simulink model "FINAL_BOARD_6437_EVM"  (Simulink 7.4)
settings: Solver=FixedStepDiscrete  StartTime=0.0  StopTime=inf  FixedStep=1/8000  RelTol=1e-3
undefined symbols (not defined in the file): M, N, SW4, sz
libraries: vipmisc x9, davincilib x6, viptransforms x3, vipconversions x3, vipgeotforms x3, dm6437evmlib x1, idelinklib_tgtpref x1, vipsrcs x1
settings Model: Creator=dsp0105  LastModifiedBy=mattwharper
settings SolverCC: PositivePriorityOrder=on
settings DataIOCC: SaveOutput=off  SaveTime=off
settings HardwareCC: ProdBitPerLong=40  ProdIntDivRoundTo=Zero  ProdEndianess=LittleEndian  ProdHWDeviceType=Texas Instruments->C6000
settings RTWCC: SystemTargetFile=ccslink_grt.tlc  GenCodeOnly=on  GenerateMakefile=off  TemplateMakefile=none  Description=Embedded IDE Link (for use with Texas Instruments(TM) Code Composer Studio(TM)) GRT code generation  ProcessScript=ccslink_grt_make_rtw_hook
settings GRTTgtLinkCCS: TargetFcnLib=ansi_tfl_table_tmw.mat  TargetFunctionLibrary=ANSI_C  UtilityFuncGeneration=Auto  ERTMultiwordTypeDef=System defined  ERTMultiwordLength=256  MultiwordLength=2048  GenerateFullHeader=on  GenerateSampleERTMain=off  GenerateTestInterfaces=off  IsPILTarget=off  ModelReferenceCompliant=on  ParMdlRefBuildCompliant=off  CompOptLevelCompliant=off  IncludeMdlTerminateFcn=on  GeneratePreprocessorConditionals=Disable all  CombineOutputUpdateFcns=off  SuppressErrorStatus=off  ERTFirstTimeCompliant=off  IncludeFileDelimiter=Auto  ERTCustomFileBanners=off  SupportAbsoluteTime=on  LogVarNameModifier=rt_  MatFileLogging=off  MultiInstanceERTCode=off  SupportNonFinite=on  SupportComplex=on  PurelyIntegerCode=off  SupportContinuousTime=on  SupportNonInlinedSFcns=on  SupportVariableSizeSignals=off  EnableShiftOperators=on  ParenthesesLevel=Nominal  PortableWordSizes=off  ModelStepFunctionPrototypeControlCompliant=off  CPPClassGenCompliant=off  AutosarCompliant=off  GenerateASAP2=off  ExtMode=off  ExtModeTransport=0  ExtModeStaticAlloc=off  ExtModeStaticAllocSize=1000000  ExtModeTesting=off  ExtModeMexFile=ext_comm  ExtModeIntrfLevel=Level1  RTWCAPISignals=off  RTWCAPIParams=off  RTWCAPIStates=off  exportCCSObj=on  ccsObjName=CCS_Obj  exportIDEObj=on  ideObjName=CCS_Obj  oldideObjName=CCS_Obj  ideObjTimeout=10  oldideObjTimeout=10  ideObjBuildTimeout=1000  oldideObjBuildTimeout=1000  ProfileGenCode=off  profileBy=Tasks  ProfileNumSamples=100  InlineDSPBlks=off  projectOptions=Custom  debugCompilerOptions="-g -d\"_DEBUG\""  releaseCompilerOptions=-o2  customCompilerOptions=-o2-q  compilerOptionsStr=-o2-q  getCompilerOptions=off  getLinkerOptions=off  systemStackSize=8192  buildAction=Build_and_execute  overrunNotificationMethod=None  overrunNotificationFcn=myfunction  oldoverrunNotificationFcn=myfunction  DiagnosticActions=warning

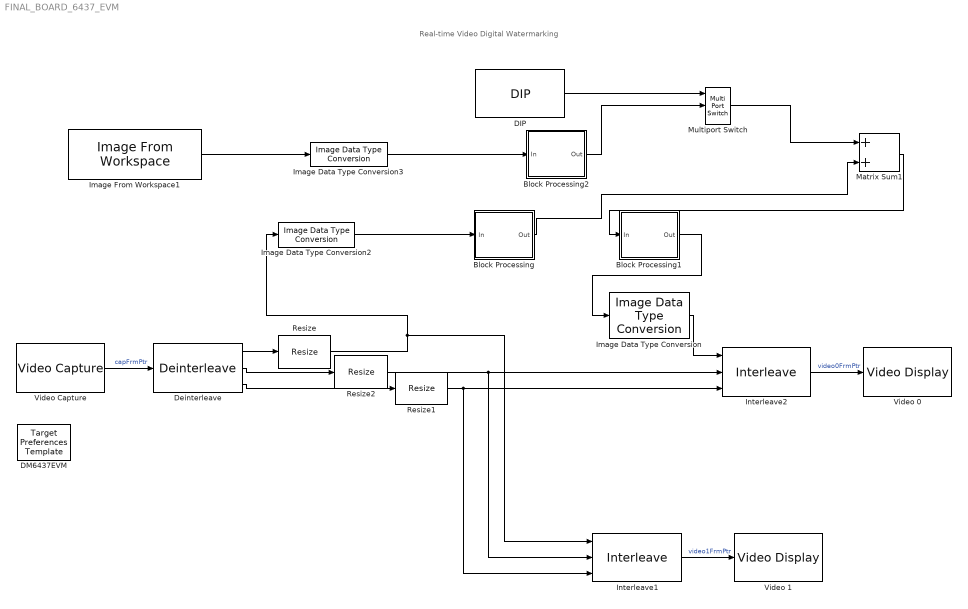
== system FINAL_BOARD_6437_EVM ==
  note: Real-time Video Digital Watermarking
  Block Processing : Subsystem  DialogController=vipDDGCreate  DialogControllerArgs=DataTag0  TreatAsAtomicUnit=on  mask(Block Processing){NumI=1, NumO=1, Blocksize={[8 8]}, Overlapsize={[0 0]}, Traverse=Row-wise}
      mask prompts: NumI "Number of inputs:"; NumO "Number of outputs:"; Blocksize "Block size:"; Overlapsize "Overlap size:"; Traverse "Order of traversing:"
      mask help:
      | Repeats a user-specified operation on submatrices of the input matrix.
      |
      | This block extracts submatrices of a user-specified size from the input matrix. It sends each submatrix to a subsystem for processing, and then reassembles each subsystem output into the output matrix.
      |
      | Use the Block size and Overlap parameters to specify the size and overlap of each submatrix in cell array format.
      mask init:
      | errmsg = vipblkblockproc(gcbh, NumI, NumO, Blocksize, Overlapsize, Traverse);
      | error(errmsg);
      settings: CopyFcn=set_param(gcb,'LinkStatus','none');
      mask Help: eval('helpview(fullfile(docroot,''toolbox'',''vipblks'',''vipblks.map''),''vipblockprocessing'')');
      mask StyleString: edit,edit,edit,edit,popup(Row-wise|Column-wise)
      mask Display: disp('Block\n Processing');
  Block Processing1 : Subsystem  DialogController=vipDDGCreate  DialogControllerArgs=DataTag2  TreatAsAtomicUnit=on  mask(Block Processing){NumI=1, NumO=1, Blocksize={[8 8]}, Overlapsize={[0 0]}, Traverse=Row-wise}
      mask prompts: NumI "Number of inputs:"; NumO "Number of outputs:"; Blocksize "Block size:"; Overlapsize "Overlap size:"; Traverse "Order of traversing:"
      mask help:
      | Repeats a user-specified operation on submatrices of the input matrix.
      |
      | This block extracts submatrices of a user-specified size from the input matrix. It sends each submatrix to a subsystem for processing, and then reassembles each subsystem output into the output matrix.
      |
      | Use the Block size and Overlap parameters to specify the size and overlap of each submatrix in cell array format.
      mask init:
      | errmsg = vipblkblockproc(gcbh, NumI, NumO, Blocksize, Overlapsize, Traverse);
      | error(errmsg);
      settings: CopyFcn=set_param(gcb,'LinkStatus','none');
      mask Help: eval('helpview(fullfile(docroot,''toolbox'',''vipblks'',''vipblks.map''),''vipblockprocessing'')');
      mask StyleString: edit,edit,edit,edit,popup(Row-wise|Column-wise)
      mask Display: disp('Block\n Processing');
  Block Processing2 : Subsystem  DialogController=vipDDGCreate  DialogControllerArgs=DataTag4  TreatAsAtomicUnit=on  mask(Block Processing){NumI=1, NumO=1, Blocksize={[8 8]}, Overlapsize={[0 0]}, Traverse=Row-wise}
      mask prompts: NumI "Number of inputs:"; NumO "Number of outputs:"; Blocksize "Block size:"; Overlapsize "Overlap size:"; Traverse "Order of traversing:"
      mask help:
      | Repeats a user-specified operation on submatrices of the input matrix.
      |
      | This block extracts submatrices of a user-specified size from the input matrix. It sends each submatrix to a subsystem for processing, and then reassembles each subsystem output into the output matrix.
      |
      | Use the Block size and Overlap parameters to specify the size and overlap of each submatrix in cell array format.
      mask init:
      | errmsg = vipblkblockproc(gcbh, NumI, NumO, Blocksize, Overlapsize, Traverse);
      | error(errmsg);
      settings: CopyFcn=set_param(gcb,'LinkStatus','none');
      mask Help: eval('helpview(fullfile(docroot,''toolbox'',''vipblks'',''vipblks.map''),''vipblockprocessing'')');
      mask StyleString: edit,edit,edit,edit,popup(Row-wise|Column-wise)
      mask Display: disp('Block\n Processing');
  DIP : dm6437evmlib/DIP  SystemSampleTime=-1  dipSwitch=SW4(0)  sampleTime=1
  DM6437EVM : idelinklib_tgtpref/Target Preferences Template  Tag=ccslinktgtpref  SystemSampleTime=-1
  Deinterleave : davincilib/Deinterleave  SystemSampleTime=-1
  Image Data Type Conversion : vipconversions/Image Data Type Conversion  outDT=uint8  isSigned=on  wordLen=16  numFracBits=0
  Image Data Type Conversion2 : vipconversions/Image Data Type Conversion  outDT=single  isSigned=on  wordLen=16  numFracBits=0
  Image Data Type Conversion3 : vipconversions/Image Data Type Conversion  outDT=single  isSigned=on  wordLen=16  numFracBits=0
  Image From Workspace1 : vipsrcs/Image From Workspace  Tag=vipblks_nd  SystemSampleTime=-1  ImageValue=h  Ts=inf  imagePorts=One multidimensional signal  ImageDataType=Inherit from 'Value'  Signed=on  WordLength=16  sdImageDataType=sfix(16)  FractionLengthMode=User-defined  FractionLength=15  OutPortLabels=R|G|B
  Interleave1 : davincilib/Interleave  SystemSampleTime=-1  outPitch=32
  Interleave2 : davincilib/Interleave  SystemSampleTime=-1  outPitch=32
  Matrix Sum1 : Sum  OutDataType=sfix(16)  OutScaling=2^-10
  Multiport Switch : MultiPortSwitch  Inputs=2  OutDataType=fixdt(1, 16)  OutScaling=2^0
  Resize : vipgeotforms/Resize  DialogController=vipDDGCreate  DialogControllerArgs=DataTag7  specify=Number of output rows and columns  rfactor=[176 128]  outCols=25  outRows=25  outRowsCols=[176 128]  interp_method=Bilinear  antialias=off  useROI=off  roiFlag=off  prodOutputMode=Binary point scaling  prodOutputWordLength=32  prodOutputFracLength=10  roundingMode=Nearest  overflowMode=on
  Resize1 : vipgeotforms/Resize  DialogController=vipDDGCreate  DialogControllerArgs=DataTag8  specify=Number of output rows and columns  rfactor=[88 128]  outCols=25  outRows=25  outRowsCols=[88 128]  interp_method=Nearest neighbor  antialias=off  useROI=off  roiFlag=off  prodOutputMode=Binary point scaling  prodOutputWordLength=32  prodOutputFracLength=10  roundingMode=Nearest  overflowMode=on
  Resize2 : vipgeotforms/Resize  DialogController=vipDDGCreate  DialogControllerArgs=DataTag9  specify=Number of output rows and columns  rfactor=[88 128]  outCols=25  outRows=25  outRowsCols=[88 128]  interp_method=Nearest neighbor  antialias=off  useROI=off  roiFlag=off  prodOutputMode=Binary point scaling  prodOutputWordLength=32  prodOutputFracLength=10  roundingMode=Nearest  overflowMode=on
  Video 0 : davincilib/Video Display  videoWindow=Video0  video0Position=[180, 0,360, 480]  video1LocSrc=Specify via dialog  video1Location=[320, 200, 152, 100]  hZoom=2x  vZoom=2x  videoEnablePort=off  videoDisplayMode=NTSC  avOutput=Composite  hExpansion=off  vExpansion=off
  Video 1 : davincilib/Video Display  videoWindow=Video1  video0Position=180, 0,360, 480]  video1LocSrc=Specify via dialog  video1Location=[0, 240, 360, 240]  hZoom=2x  vZoom=2x  videoEnablePort=off  videoDisplayMode=NTSC  avOutput=Composite  hExpansion=off  vExpansion=off
  Video Capture : davincilib/Video Capture  videoCaptureMode=NTSC  avInput=Composite  sampleTime=-1
  wires:
  Video Capture/1 -> Deinterleave/1  "capFrmPtr"
  Interleave2/1 -> Video 0/1  "video0FrmPtr"
  Image Data Type Conversion/1 -> Interleave2/1
  Deinterleave/3 -> Resize1/1
  Deinterleave/2 -> Resize2/1
  Deinterleave/1 -> Resize/1
  Block Processing1/1(Out) -> Image Data Type Conversion/1
  Interleave1/1 -> Video 1/1  "video1FrmPtr"
  Multiport Switch/1 -> Matrix Sum1/1
  Block Processing2/1(Out) -> Multiport Switch/2
  DIP/1 -> Multiport Switch/1
  Matrix Sum1/1 -> Block Processing1/1(In)
  Block Processing/1(Out) -> Matrix Sum1/2
  Image From Workspace1/1 -> Image Data Type Conversion3/1
  Image Data Type Conversion3/1 -> Block Processing2/1(In)
  Image Data Type Conversion2/1 -> Block Processing/1(In)
  Resize/1 -> Interleave1/1, Image Data Type Conversion2/1
  Resize2/1 -> Interleave2/2, Interleave1/2
  Resize1/1 -> Interleave2/3, Interleave1/3

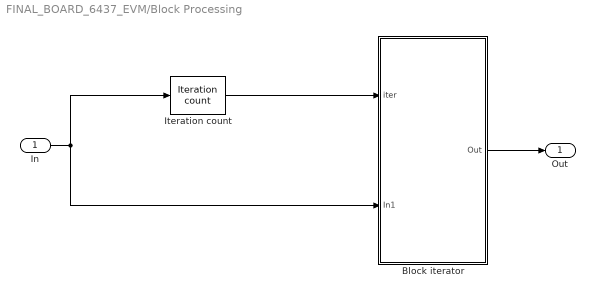
== system FINAL_BOARD_6437_EVM/Block Processing ==
  In : Inport  OutDataType=sfix(16)  OutScaling=2^0
  Block iterator : Subsystem
      settings: CopyFcn=set_param(gcb,'ReferenceBlock','');
  Iteration count : vipmisc/Iteration count  blksize=Blocksize{1}  ovlpsize=Overlapsize{1}
  Out : Outport  OutDataType=sfix(16)  OutScaling=2^0
  wires:
  Iteration count/1 -> Block iterator/1(iter)
  In/1 -> Iteration count/1, Block iterator/2(In1)
  Block iterator/1(Out) -> Out/1

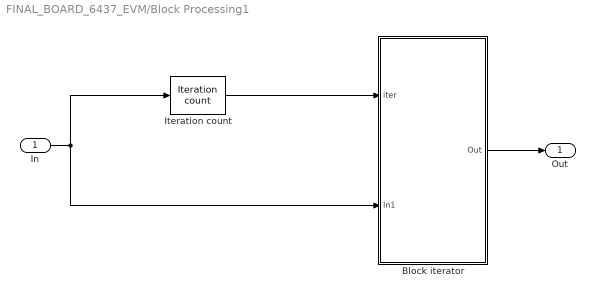
== system FINAL_BOARD_6437_EVM/Block Processing1 ==
  In : Inport  OutDataType=sfix(16)  OutScaling=2^0
  Block iterator : Subsystem
      settings: CopyFcn=set_param(gcb,'ReferenceBlock','');
  Iteration count : vipmisc/Iteration count  blksize=Blocksize{1}  ovlpsize=Overlapsize{1}
  Out : Outport  OutDataType=sfix(16)  OutScaling=2^0
  wires:
  Iteration count/1 -> Block iterator/1(iter)
  In/1 -> Iteration count/1, Block iterator/2(In1)
  Block iterator/1(Out) -> Out/1

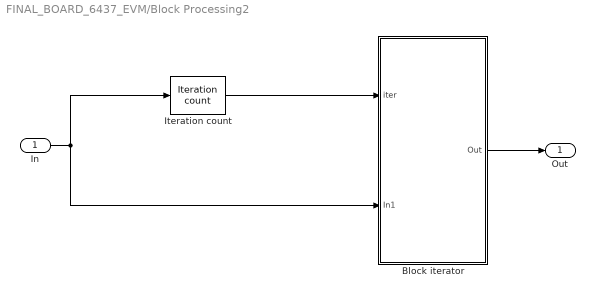
== system FINAL_BOARD_6437_EVM/Block Processing2 ==
  In : Inport  OutDataType=sfix(16)  OutScaling=2^0
  Block iterator : Subsystem
      settings: CopyFcn=set_param(gcb,'ReferenceBlock','');
  Iteration count : vipmisc/Iteration count  blksize=Blocksize{1}  ovlpsize=Overlapsize{1}
  Out : Outport  OutDataType=sfix(16)  OutScaling=2^0
  wires:
  Iteration count/1 -> Block iterator/1(iter)
  In/1 -> Iteration count/1, Block iterator/2(In1)
  Block iterator/1(Out) -> Out/1

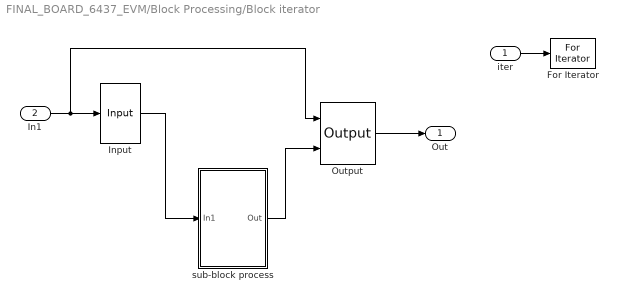
== system FINAL_BOARD_6437_EVM/Block Processing/Block iterator ==
  iter : Inport  OutDataType=sfix(16)  OutScaling=2^0
  In1 : Inport  Port=2  OutDataType=sfix(16)  OutScaling=2^0
  For Iterator : ForIterator  IterationSource=external  IterationLimit=(sz(1)/M)*(sz(2)/N)  ShowIterationPort=off  IndexMode=Zero-based  IterationVariableDataType=double
  Input : vipmisc/Input  SystemSampleTime=-1  Blocksize=Blocksize{1}  Overlapsize=Overlapsize{1}  tverse=Row-wise
  Output : vipmisc/Output  SystemSampleTime=-1  Blocksize=Blocksize{1}  Overlapsize=Overlapsize{1}  tverse=Row-wise
  sub-block process : Subsystem
  Out : Outport  OutDataType=sfix(16)  OutScaling=2^0
  wires:
  iter/1 -> For Iterator/1
  In1/1 -> Output/1, Input/1
  Output/1 -> Out/1
  sub-block process/1(Out) -> Output/2
  Input/1 -> sub-block process/1(In1)

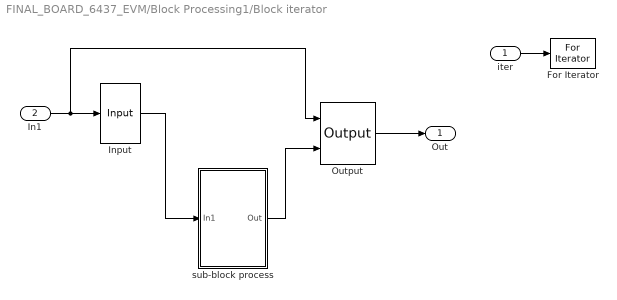
== system FINAL_BOARD_6437_EVM/Block Processing1/Block iterator ==
  iter : Inport  OutDataType=sfix(16)  OutScaling=2^0
  In1 : Inport  Port=2  OutDataType=sfix(16)  OutScaling=2^0
  For Iterator : ForIterator  IterationSource=external  IterationLimit=(sz(1)/M)*(sz(2)/N)  ShowIterationPort=off  IndexMode=Zero-based  IterationVariableDataType=double
  Input : vipmisc/Input  SystemSampleTime=-1  Blocksize=Blocksize{1}  Overlapsize=Overlapsize{1}  tverse=Row-wise
  Output : vipmisc/Output  SystemSampleTime=-1  Blocksize=Blocksize{1}  Overlapsize=Overlapsize{1}  tverse=Row-wise
  sub-block process : Subsystem
  Out : Outport  OutDataType=sfix(16)  OutScaling=2^0
  wires:
  iter/1 -> For Iterator/1
  In1/1 -> Output/1, Input/1
  Output/1 -> Out/1
  sub-block process/1(Out) -> Output/2
  Input/1 -> sub-block process/1(In1)

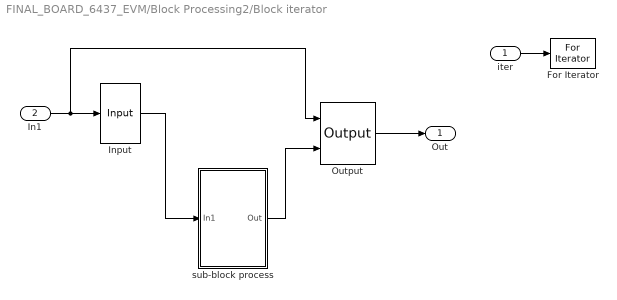
== system FINAL_BOARD_6437_EVM/Block Processing2/Block iterator ==
  iter : Inport  OutDataType=sfix(16)  OutScaling=2^0
  In1 : Inport  Port=2  OutDataType=sfix(16)  OutScaling=2^0
  For Iterator : ForIterator  IterationSource=external  IterationLimit=(sz(1)/M)*(sz(2)/N)  ShowIterationPort=off  IndexMode=Zero-based  IterationVariableDataType=double
  Input : vipmisc/Input  SystemSampleTime=-1  Blocksize=Blocksize{1}  Overlapsize=Overlapsize{1}  tverse=Row-wise
  Output : vipmisc/Output  SystemSampleTime=-1  Blocksize=Blocksize{1}  Overlapsize=Overlapsize{1}  tverse=Row-wise
  sub-block process : Subsystem
  Out : Outport  OutDataType=sfix(16)  OutScaling=2^0
  wires:
  iter/1 -> For Iterator/1
  In1/1 -> Output/1, Input/1
  Output/1 -> Out/1
  sub-block process/1(Out) -> Output/2
  Input/1 -> sub-block process/1(In1)

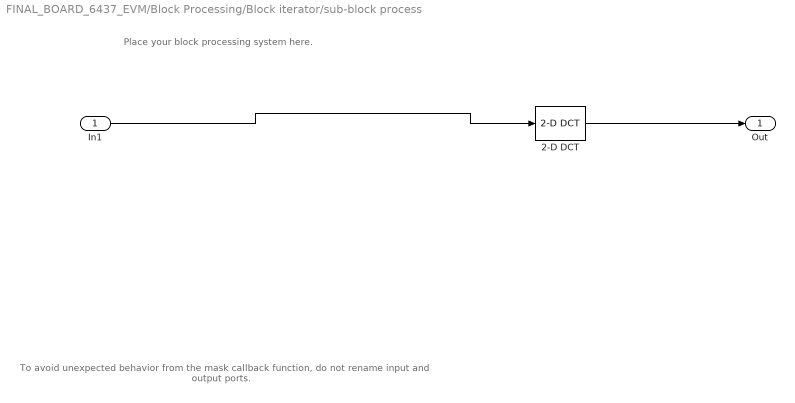
== system FINAL_BOARD_6437_EVM/Block Processing/Block iterator/sub-block process ==
  note: To avoid unexpected behavior from the mask
      | callback function, do not rename input and output ports.
  note: Place your block
      | processing system here.
  In1 : Inport  OutDataType=sfix(16)  OutScaling=2^0
  2-D DCT : viptransforms/2-D DCT  DialogController=dspDDGCreate  DialogControllerArgs=DataTag1  CompMethod=Table lookup  Dimension=0  TableOpt=Speed  BitRevOrder=off  SkipNorm=off  roundingMode=Floor  overflowMode=off
  Out : Outport  OutDataType=sfix(16)  OutScaling=2^0
  wires:
  2-D DCT/1 -> Out/1
  In1/1 -> 2-D DCT/1

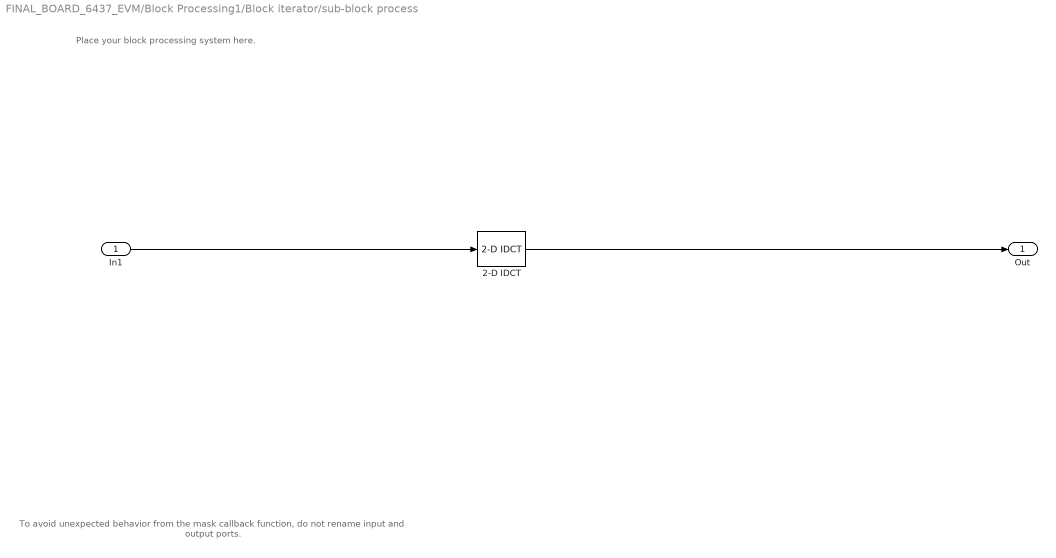
== system FINAL_BOARD_6437_EVM/Block Processing1/Block iterator/sub-block process ==
  note: To avoid unexpected behavior from the mask
      | callback function, do not rename input and output ports.
  note: Place your block
      | processing system here.
  In1 : Inport  OutDataType=sfix(16)  OutScaling=2^0
  2-D IDCT : viptransforms/2-D IDCT  DialogController=dspDDGCreate  DialogControllerArgs=DataTag3  CompMethod=Table lookup  Dimension=0  TableOpt=Speed  BitRevOrder=off  SkipNorm=off  roundingMode=Floor  overflowMode=off
  Out : Outport  OutDataType=sfix(16)  OutScaling=2^0
  wires:
  2-D IDCT/1 -> Out/1
  In1/1 -> 2-D IDCT/1

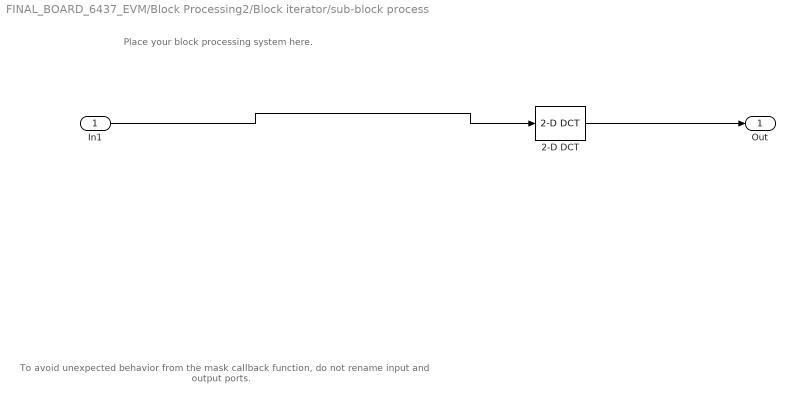
== system FINAL_BOARD_6437_EVM/Block Processing2/Block iterator/sub-block process ==
  note: To avoid unexpected behavior from the mask
      | callback function, do not rename input and output ports.
  note: Place your block
      | processing system here.
  In1 : Inport  OutDataType=sfix(16)  OutScaling=2^0
  2-D DCT : viptransforms/2-D DCT  DialogController=dspDDGCreate  DialogControllerArgs=DataTag5  CompMethod=Table lookup  Dimension=0  TableOpt=Speed  BitRevOrder=off  SkipNorm=off  roundingMode=Floor  overflowMode=off
  Out : Outport  OutDataType=sfix(16)  OutScaling=2^0
  wires:
  2-D DCT/1 -> Out/1
  In1/1 -> 2-D DCT/1
